simulink model "test"  (R2016b)
settings: Solver=VariableStepAuto  StartTime=0.0  StopTime=10.0  RelTol=1e-3
settings Model: Creator=Biscuit  LastModifiedBy=Biscuit

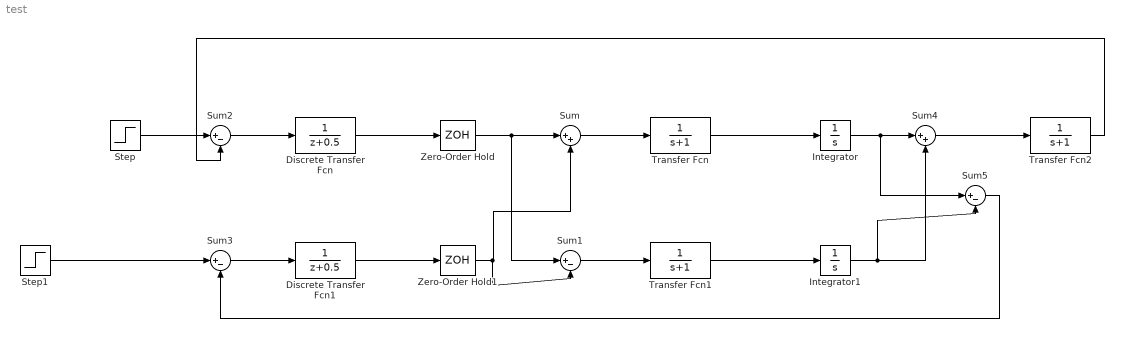
== system test ==
  Discrete Transfer Fcn : DiscreteTransferFcn
  Discrete Transfer Fcn1 : DiscreteTransferFcn
  Integrator : Integrator
  Integrator1 : Integrator
  Step : Step  SampleTime=0
  Step1 : Step  SampleTime=0
  Sum : Sum  Inputs=|++
  Sum{1..3,5} (4 alike) : Sum  Inputs=|+-
  Sum4 : Sum  Inputs=|++
  Transfer Fcn : TransferFcn  Denominator=[1 1]
  Transfer Fcn1 : TransferFcn  Denominator=[1 1]
  Transfer Fcn2 : TransferFcn  Denominator=[1 1]
  Zero-Order Hold : ZeroOrderHold  SampleTime=-1
  Zero-Order Hold1 : ZeroOrderHold  SampleTime=-1
  wires:
  Discrete Transfer Fcn/1 -> Zero-Order Hold/1
  Discrete Transfer Fcn1/1 -> Zero-Order Hold1/1
  Sum/1 -> Transfer Fcn/1
  Zero-Order Hold/1 -> Sum1/1, Sum/1
  Sum1/1 -> Transfer Fcn1/1
  Zero-Order Hold1/1 -> Sum1/2, Sum/2
  Sum2/1 -> Discrete Transfer Fcn/1
  Step/1 -> Sum2/1
  Sum3/1 -> Discrete Transfer Fcn1/1
  Step1/1 -> Sum3/1
  Transfer Fcn/1 -> Integrator/1
  Transfer Fcn1/1 -> Integrator1/1
  Sum4/1 -> Transfer Fcn2/1
  Transfer Fcn2/1 -> Sum2/2
  Integrator/1 -> Sum5/1, Sum4/1
  Integrator1/1 -> Sum5/2, Sum4/2
  Sum5/1 -> Sum3/2
